simulink model "HW1_2c"  (R2021b)
settings: Solver=VariableStepAuto  StartTime=0.0  StopTime=10.0  RelTol=1e-3
undefined symbols (not defined in the file): kd, kp, t0
settings Model: Creator=capn  LastModifiedBy=capn
settings SolverCC: AlgebraicLoopSolver=TrustRegion
settings DataIOCC: ReturnWorkspaceOutputs=off
settings DebuggingCC: SFMachineParentedDataDiag=warning  ArithmeticOperatorsInVariantConditions=warning
settings SFSimCC: SimUseLocalCustomCode=off  CustomCodeUndefinedFunction=UseInterfaceOnly
settings RTWCC: RTWUseLocalCustomCode=off
settings CodeAppCC: StateflowObjectComments=on

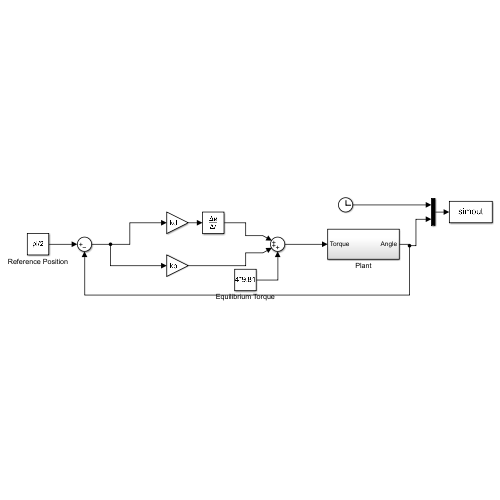
[thumbnail: Simulink's stored preview of the top-level diagram]
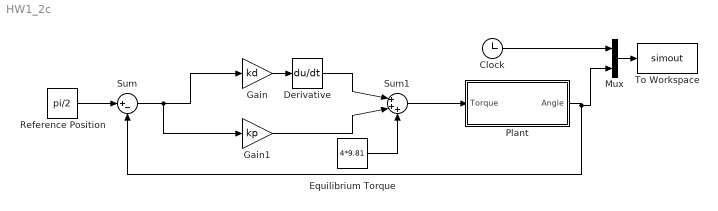
== system HW1_2c ==
  Clock : Clock
  Derivative : Derivative  CoefficientInTFapproximation=0
  Equilibrium Torque : Constant  Value=4*9.81
  Gain : Gain  Gain=kd
  Gain1 : Gain  Gain=kp
  Mux : Mux  Inputs=2
  Plant : Subsystem
  Reference Position : Constant  Value=pi/2
  Sum : Sum  Inputs=|+-
  Sum1 : Sum  Inputs=|+++
  To Workspace : ToWorkspace  VariableName=simout  SampleTime=-1
  wires:
  Gain/1 -> Derivative/1
  Reference Position/1 -> Sum/1
  Sum1/1 -> Plant/1(Torque)
  Derivative/1 -> Sum1/1
  Gain1/1 -> Sum1/2
  Sum/1 -> Gain1/1, Gain/1
  Plant/1(Angle) -> Mux/2, Sum/2
  Clock/1 -> Mux/1
  Mux/1 -> To Workspace/1
  Equilibrium Torque/1 -> Sum1/3

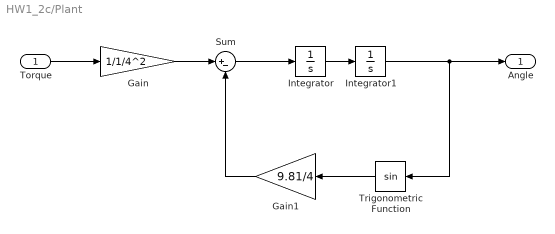
== system HW1_2c/Plant ==
  Torque : Inport
  Gain : Gain  Gain=1/1/4^2
  Gain1 : Gain  Gain=9.81/4
  Integrator : Integrator
  Integrator1 : Integrator  InitialCondition=t0
  Sum : Sum  Inputs=|+-
  Trigonometric Function : Trigonometry
  Angle : Outport  VectorParamsAs1DForOutWhenUnconnected=off
  wires:
  Torque/1 -> Gain/1
  Gain/1 -> Sum/1
  Sum/1 -> Integrator/1
  Integrator/1 -> Integrator1/1
  Integrator1/1 -> Trigonometric Function/1, Angle/1
  Trigonometric Function/1 -> Gain1/1
  Gain1/1 -> Sum/2
